simulink model "RefModel_compass_18b"  (R2019b)
settings: Solver=FixedStepDiscrete  StartTime=0.0  StopTime=10  RelTol=1e-3
libraries: simulink x1, aerolibgravity2 x1
settings Model: Creator=sl  LastModifiedBy=a4327
settings OptimizationCC: DefaultParameterBehavior=Inlined  EnhancedBackFolding=on  PassReuseOutputArgsAs=Individual arguments  ZeroExternalMemoryAtStartup=off  ZeroInternalMemoryAtStartup=off  OptimizeBlockOrder=speed  DifferentSizesBufferReuse=on  OptimizationCustomize=off  EfficientTunableParamExpr=on
settings DebuggingCC: ParameterTunabilityLossMsg=error  ArithmeticOperatorsInVariantConditions=warning
settings SFSimCC: MATLABDynamicMemAlloc=off  CustomCodeUndefinedFunction=UseInterfaceOnly
settings RTWCC: SystemTargetFile=ert.tlc  TemplateMakefile=ert_default_tmf  GenerateReport=on  IncludeHyperlinkInReport=on  LaunchReport=on  GenerateTraceInfo=on  GenerateTraceReport=on  GenerateTraceReportSl=on  GenerateTraceReportSf=on  GenerateTraceReportEml=on
settings CodeAppCC: ForceParamTrailComments=on  IgnoreCustomStorageClasses=off  OperatorAnnotations=on  SimulinkDataObjDesc=on  SFDataObjDesc=on  InsertBlockDesc=on
settings ERTTargetCC: TargetLangStandard=C99 (ISO)  GenerateSampleERTMain=on  InlinedParameterPlacement=NonHierarchical  ERTCustomFileTemplate=example_file_process.tlc

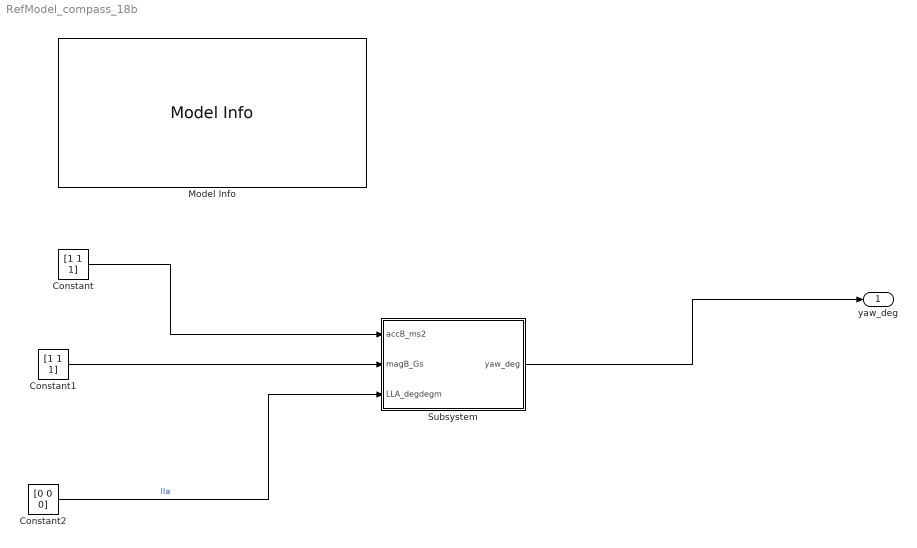
== system RefModel_compass_18b ==
  Constant : Constant  Value=[1 1 1]
  Constant1 : Constant  Value=[1 1 1]
  Constant2 : Constant  Value=[0 0 0]
  Model Info : simulink/Model-Wide Utilities/Model Info  Frame=on  DisplayStringWithTags=|  HorizontalTextAlignment=Left  LeftAlignmentValue=0.02
      | %<ModelVersion>
      | %<LastModificationDate>
      | 
      | Body Coordinate: forward - right - down
      | Navigation Coordinate: NED
      | 
      | input:
      | 	accB_ms2:  1x3  m/s^2
      | 	magB_Gs:   1x3  Gs
      | 	LLA_degdegm(lat,lon,height): 1x3 deg,deg,m  
      | output:
      | 	yaw_deg: 1x1 deg
  Subsystem : Subsystem
  yaw_deg : Outport
  wires:
  Constant/1 -> Subsystem/1(accB_ms2)
  Constant1/1 -> Subsystem/2(magB_Gs)
  Constant2/1 -> Subsystem/3(LLA_degdegm)  "lla"
  Subsystem/1(yaw_deg) -> yaw_deg/1

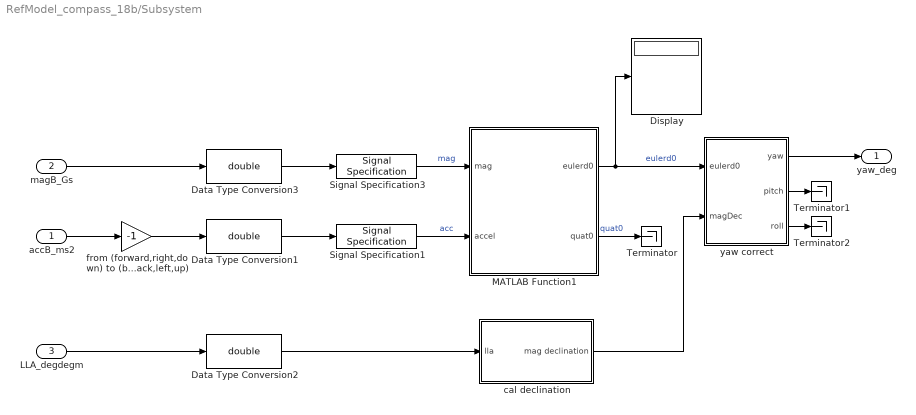
== system RefModel_compass_18b/Subsystem ==
  accB_ms2 : Inport  PortDimensions=[1,3]
  magB_Gs : Inport  Port=2  PortDimensions=[1,3]
  LLA_degdegm : Inport  Port=3  PortDimensions=[1,3]
  Data Type Conversion1 : DataTypeConversion  OutDataTypeStr=double
  Data Type Conversion2 : DataTypeConversion  OutDataTypeStr=double
  Data Type Conversion3 : DataTypeConversion  OutDataTypeStr=double
  Display : Display
  MATLAB Function1 : MATLAB Function  TreatAsAtomicUnit=on
  Signal Specification1 : SignalSpecification  Dimensions=[1,3]
  Signal Specification3 : SignalSpecification  Dimensions=[1,3]
  Terminator : Terminator
  Terminator1 : Terminator
  Terminator2 : Terminator
  cal declination : Subsystem
  from (forward,right,down) to (back,left,up) : Gain  Gain=-1
  yaw correct : Subsystem
  yaw_deg : Outport
  wires:
  MATLAB Function1/2(quat0) -> Terminator/1  "quat0"
  from (forward,right,down) to (back,left,up)/1 -> Data Type Conversion1/1
  MATLAB Function1/1(eulerd0) -> Display/1, yaw correct/1(eulerd0)  "eulerd0"
  Signal Specification3/1 -> MATLAB Function1/1(mag)  "mag"
  yaw correct/2(pitch) -> Terminator1/1
  Data Type Conversion1/1 -> Signal Specification1/1
  Data Type Conversion3/1 -> Signal Specification3/1
  yaw correct/1(yaw) -> yaw_deg/1
  magB_Gs/1 -> Data Type Conversion3/1
  accB_ms2/1 -> from (forward,right,down) to (back,left,up)/1
  yaw correct/3(roll) -> Terminator2/1
  Signal Specification1/1 -> MATLAB Function1/2(accel)  "acc"
  cal declination/1(mag declination) -> yaw correct/2(magDec)
  Data Type Conversion2/1 -> cal declination/1(lla)
  LLA_degdegm/1 -> Data Type Conversion2/1

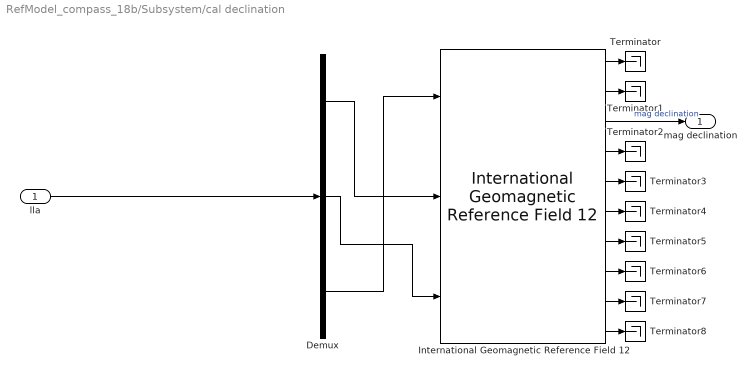
== system RefModel_compass_18b/Subsystem/cal declination ==
  lla : Inport
  Demux : Demux  Outputs=3
  International Geomagnetic Reference Field 12 : aerolibgravity2/International Geomagnetic Reference Field 12  units=Metric (MKS)  time_in=off  month=December  day=20  year=2019  action=None  sv_out=on
      settings: SourceProductName=Aerospace Blockset  SourceProductBaseCode=AE
  Terminator{,1..8} (9 alike) : Terminator
  mag declination : Outport
  wires:
  Demux/3 -> International Geomagnetic Reference Field 12/1
  Demux/1 -> International Geomagnetic Reference Field 12/2
  International Geomagnetic Reference Field 12/9 -> Terminator7/1
  International Geomagnetic Reference Field 12/10 -> Terminator8/1
  International Geomagnetic Reference Field 12/4 -> Terminator2/1
  International Geomagnetic Reference Field 12/1 -> Terminator/1
  Demux/2 -> International Geomagnetic Reference Field 12/3
  International Geomagnetic Reference Field 12/2 -> Terminator1/1
  International Geomagnetic Reference Field 12/3 -> mag declination/1  "mag declination"
  International Geomagnetic Reference Field 12/5 -> Terminator3/1
  International Geomagnetic Reference Field 12/6 -> Terminator4/1
  International Geomagnetic Reference Field 12/8 -> Terminator6/1
  International Geomagnetic Reference Field 12/7 -> Terminator5/1
  lla/1 -> Demux/1

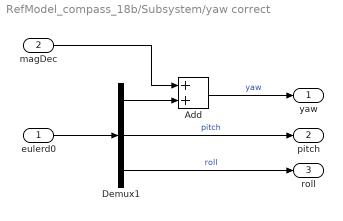
== system RefModel_compass_18b/Subsystem/yaw correct ==
  eulerd0 : Inport
  magDec : Inport  Port=2
  Add : Sum
  Demux1 : Demux  Outputs=3
  yaw : Outport
  pitch : Outport  Port=2
  roll : Outport  Port=3
  wires:
  magDec/1 -> Add/1
  eulerd0/1 -> Demux1/1
  Demux1/2 -> pitch/1  "pitch"
  Demux1/3 -> roll/1  "roll"
  Demux1/1 -> Add/2
  Add/1 -> yaw/1  "yaw"

== matlab function RefModel_compass_18b/Subsystem/MATLAB Function1 ==
  data: mag input; accel input; eulerd0 output; quat0 output
function [eulerd0,quat0] = compass(mag,accel)
    quat0 = zeros(1,4);
    eulerd0 = zeros(1,3);
    temp=ecompass(accel,mag);
    quat0 = compact(temp);
%     eulerd0 = eulerd(quat0);
    eulerd0 = to_euler(quat0);
    
end


function eout = eulerd(quat)
% rotate 'ZYX'
qa = quat(1);
qb = quat(2);
qc = quat(3);
qd = quat(4);
the1 = 1;
the2 = 2;

tmp = qb.*qd.*the2 - qa.*qc.*the2;
if tmp > the1
    tmp = the1;
elseif tmp < -the1
    tmp = -the1;
end
% tmp(tmp > the1) = the1;
% tmp(tmp < -the1) = -the1;
b = -asin(tmp);
a = atan2((qa.*qd.*the2 + qb.*qc.*the2),(qa.^2.*the2 - the1 + qb.^2.*the2));
c = atan2((qa.*qb.*the2 + qc.*qd.*the2),(qa.^2.*the2 - the1 + qd.^2.*the2));
eout = [a b c]*180/pi;
end

% 
% function [eulerd0,quat0] = compass(i,accel,mag,imuUpdateFs,magUpdateFs)
%     fs = imuUpdateFs;
%     quat0 = zeros(1,4);
%     eulerd0 = zeros(1,3);
%     if rem(i,fs/magUpdateFs) == 0 && i ~= 1
%         quat0 = compact(ecompass(accel,mag));
%         eulerd0 = eulerd(quat0);
%     end
% end
